simulink model "idhp_model_heart_realtime_syn"  (R2014a)
settings: Solver=FixedStepDiscrete  StartTime=0.0  StopTime=100  FixedStep=0.01  RelTol=1e-3
settings Model: Creator=alexandru  LastModifiedBy=alexandru
settings DataIOCC: LimitDataPoints=off  SaveOutput=off  SignalLogging=off  DSMLogging=off  SaveTime=off
settings HardwareCC: TargetBitPerLong=64  TargetBitPerPointer=64  TargetLongLongMode=on  TargetIntDivRoundTo=Zero  TargetEndianess=LittleEndian  TargetWordSize=64  TargetHWDeviceType=MATLAB Host  ProdEqTarget=off
settings RTWCC: SystemTargetFile=rsim.tlc  GenCodeOnly=on  PackageGeneratedCodeAndArtifacts=on  PackageName=idhp_model_heart_realtime  TemplateMakefile=rsim_default_tmf  Description=Rapid Simulation Target  ProcessScript=rsim_make_rtw_hook
settings RSimTargetCC: ERTMultiwordTypeDef=System defined  ERTMultiwordLength=256  EnableShiftOperators=on

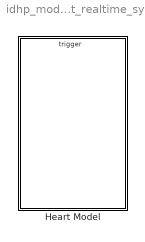
== system idhp_model_heart_realtime_syn ==
  Heart Model : Stateflow chart  Priority=1  TreatAsAtomicUnit=on

== stateflow chart idhp_model_heart_realtime_syn/Heart Model ==
  state Pacemaker
    state LRI [parallel]
      settings: executionOrder=4
      state LRI
      state ASensed
      Pacemaker.LRI.LRI -> Pacemaker.LRI.LRI [order 2] : after(PM_TLRI-PM_TAVI,msec)
          | {send(AP,AVI);send(AP,PaceLedAtrium);
          | SWrite(0x33);SWrite(0x35);}
      Pacemaker.LRI.LRI -> ASensed [order 3] : AS
      ASensed -> Pacemaker.LRI.LRI : RLRI
      Pacemaker.LRI.LRI -> Pacemaker.LRI.LRI [order 1] : RLRI
      (default) -> Pacemaker.LRI.LRI
    state URI [parallel]
      settings: executionOrder=5
      state URI
      state q1
      Pacemaker.URI.URI -> Pacemaker.URI.URI [order 1] : RURI
      Pacemaker.URI.URI -> Pacemaker.URI.q1 [order 2] : after(PM_TURI,msec){SWrite(0x36);}
      (default) -> Pacemaker.URI.URI
      Pacemaker.URI.q1 -> Pacemaker.URI.URI : {send(IncrClk,AVI);}
    state AVI [parallel]
      settings: executionOrder=1
      state Idle0
      state AVI0
      state WaitURI
      state Idle1
      state AVI1
      WaitURI -> Idle0 [order 1] : VS{send(RURI,URI);}
      AVI0 -> Idle0 [order 3] : VS{send(RURI,URI);}
      Idle0 -> AVI0 [order 2] : AP{send(RTAVI,TAVIcmp);}
      (default) -> Idle0
      AVI0 -> WaitURI [order 2] : TAVI
      Idle0 -> AVI0 [order 3] : AS{send(RTAVI,TAVIcmp);}
      AVI1 -> Idle0 [order 2] : TAVI{
          | send(RLRI,LRI);
          | send(VP,VRP);
          | send(VP,PVARP);
          | send(RURI,URI);
          | send(VP,PaceLedVentricle);
          | SWrite(0x34);}
      AVI1 -> Idle0 [order 1] : VS{send(RURI,URI);}
      WaitURI -> Idle0 [order 2] : IncrClk{
          | send(RLRI,LRI);
          | send(VP,VRP);
          | send(VP,PVARP);
          | send(VP,PaceLedVentricle);
          | SWrite(0x34);}
      AVI0 -> AVI1 [order 1] : IncrClk
      Idle0 -> Idle1 [order 1] : IncrClk
      Idle1 -> AVI1 [order 2] : AP{send(RTAVI,TAVIcmp);}
      Idle1 -> AVI1 [order 1] : AS{send(RTAVI,TAVIcmp);}
    state VRP [parallel]
      settings: executionOrder=2
      state Idle
      state VRP
      state Vsig
      Pacemaker.VRP.VRP -> Pacemaker.VRP.Idle : after(PM_TVRP,msec){SWrite(0x38);}
      (default) -> Pacemaker.VRP.Idle
      Pacemaker.VRP.Idle -> Pacemaker.VRP.VRP [order 2] : VP
      Vsig -> Pacemaker.VRP.Idle : {send(RLRI, LRI);
          | send(VS, AVI);
          | send(VS, PVARP);}
      Pacemaker.VRP.Idle -> Vsig [order 1] : Vget
    state TAVIcmp [parallel]
      settings: executionOrder=6
      state q0
      state q1
      q0 -> Pacemaker.TAVIcmp.q1 : after(PM_TAVI,msec)
          | {send(TAVI,AVI);
          | SWrite(0x37);}
      Pacemaker.TAVIcmp.q1 -> q0 : RTAVI
      (default) -> Pacemaker.TAVIcmp.q1
    state PVARP [parallel]
      settings: executionOrder=3
      state Idle
      state PVAB
      state Asig
      state PVARP
      Pacemaker.PVARP.Idle -> PVAB [order 3] : VP
      Pacemaker.PVARP.Idle -> PVAB [order 2] : VS
      (default) -> Pacemaker.PVARP.Idle
      Pacemaker.PVARP.PVARP -> Pacemaker.PVARP.Idle : after(PM_TPVARP-...
          | PM_TPVAB,msec)
          | {SWrite(0x39);}
      Asig -> Pacemaker.PVARP.Idle : {send(AS,LRI);
          | send(AS,AVI);
          | send(AS,TAVIcmp);}
      Pacemaker.PVARP.Idle -> Asig [order 1] : Aget
      PVAB -> Pacemaker.PVARP.PVARP : after(PM_TPVAB,msec)
          | {SWrite(0x3A);}
    state SerialPort [parallel]
      settings: executionOrder=7
      state NoData
      state Receive
      Receive -> NoData [order 1] : [bufs1==0x31]{send(Aget, PVARP);}
      (default) -> NoData
      Receive -> NoData [order 2] : [bufs1==0x32]{send(Vget, VRP);}
      NoData -> Receive : SREC
          | {bufs1 = SReceive();}
    state PaceLedAtrium [parallel]
      settings: executionOrder=8
      state Off
      state On
      (default) -> Pacemaker.PaceLedAtrium.Off : {dW(12, 0);}
      Pacemaker.PaceLedAtrium.On -> Pacemaker.PaceLedAtrium.Off : after(2, msec)
          | {dW(12, 0);}
      Pacemaker.PaceLedAtrium.Off -> Pacemaker.PaceLedAtrium.On : AP
          | {dW(12, 1);}
    state PaceLedVentricle [parallel]
      settings: executionOrder=9
      state Off
      state On
      (default) -> Pacemaker.PaceLedVentricle.Off : {dW(11, 0);}
      Pacemaker.PaceLedVentricle.On -> Pacemaker.PaceLedVentricle.Off : after(2, msec)
          | {dW(11, 0);}
      Pacemaker.PaceLedVentricle.Off -> Pacemaker.PaceLedVentricle.On : VP
          | {dW(11, 1);}
  (default) -> Pacemaker
  data: buf function_output double; stat function_output double; h function_input double; stat function_output double; c function_input double; value function_input double; stat function_output double; port function_input double; value function_input double; BAUDRATE local uint32 =57600; parid local uint16; parval local double; bufs2 local uint8; bufs1 local uint8; bufs3 local uint8; bufs4 local uint8; bufs5 local uint8; PM_TAVI local uint32 =150; PM_TLRI local uint32 =1000; PM_TPVAB local uint32 =50; PM_TPVARP local uint32 =250; PM_TURI local uint32 =500; PM_TVRP local uint32 =320; tmp16 local uint16; tmp32 local uint32; value local uint32
  data BAUDRATE settings: description=Cosmos
  events: AP local EITHER_EDGE_EVENT; VP local EITHER_EDGE_EVENT; AS local RISING_EDGE_EVENT; VS local RISING_EDGE_EVENT; Aget local EITHER_EDGE_EVENT; Vget local EITHER_EDGE_EVENT; RLRI local FUNCTION_CALL_EVENT; TAVI local FUNCTION_CALL_EVENT; RTAVI local FUNCTION_CALL_EVENT; RURI local FUNCTION_CALL_EVENT; IncrClk local FUNCTION_CALL_EVENT; SREC input FUNCTION_CALL_EVENT
  function buf  = SReceive:
    | function buf  = SReceive()
    |     buf = 0;
    | end
  function stat  = SWrite(h):
    | function stat  = SWrite(h)
    | stat = 0;
    | end
  function stat  = SetParameters(c, value):
    | function stat  = SetParameters(c, value)
    | stat  = 0;
    | end
  function stat  = dW(port, value):
    | function stat  = dW(port, value)
    | stat  = 0;
    | digitalWrite(port, value);
    | end
